simulink model "ROTATIONAL_DYNAMICS_old"  (R2024b)
settings: Solver=VariableStepAuto  StartTime=0.0  StopTime=20  RelTol=1e-3
values from neighbouring files (symbols this model uses):
  A_alt_aug = [A_alt, zeros(size(A_alt,1),1); -C_alt, 0]    [STATE_SPACE_CALCULATIONS_v2.m]
  A_altitude = [ ... (first row only)    [STATE_SPACE_CALCULATIONS.m]
  B_alt_aug = [B_alt; 0]    [STATE_SPACE_CALCULATIONS_v2.m]
  B_altitude = [ ... (first row only)    [STATE_SPACE_CALCULATIONS.m]
  C_alt_aug = [C_alt 0]    [STATE_SPACE_CALCULATIONS_v2.m]
  C_altitude = [1, 0, 0]    [STATE_SPACE_CALCULATIONS.m]
  D_alt_aug = D_alt    [STATE_SPACE_CALCULATIONS_v2.m]
  D_altitude = [0]    [STATE_SPACE_CALCULATIONS.m]
  K_alt_aug = lqr(A_alt_aug, B_alt_aug, Q_alt_aug, R_alt)    [STATE_SPACE_CALCULATIONS_v2.m]
  K_altitude = lqr(A_altitude, B_altitude, Q_altitude, R_altitude)    [STATE_SPACE_CALCULATIONS.m]
settings Model: Creator=hazza  LastModifiedBy=hazza

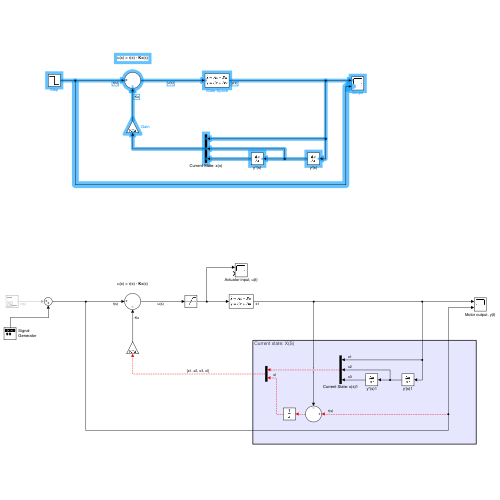
[thumbnail: Simulink's stored preview of the top-level diagram]
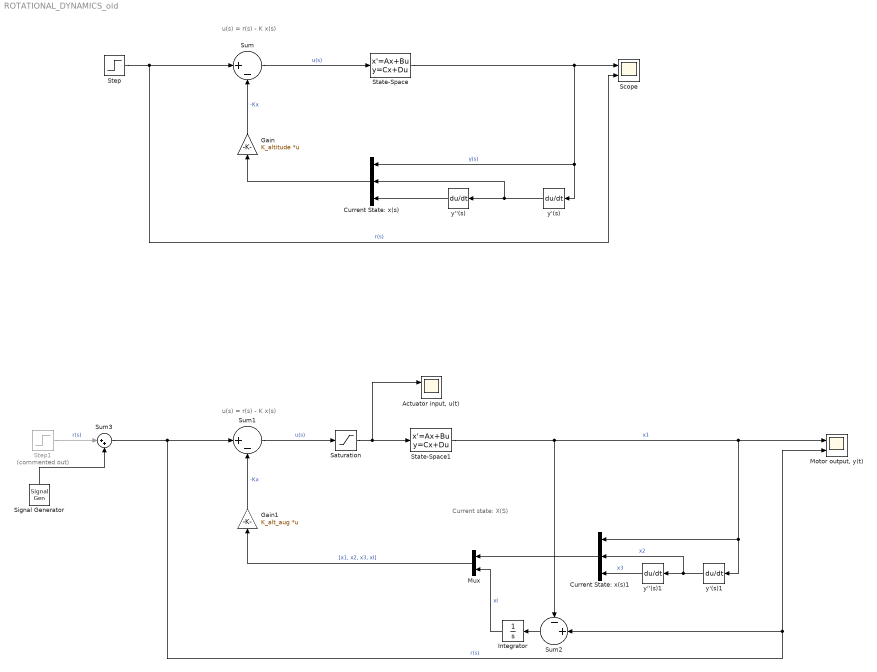
== system ROTATIONAL_DYNAMICS_old ==
  note: Current state: X(S)
  note: u(s) = r(s) - K x(s)
  note: u(s) = r(s) - K x(s)
  "Actuator input, u(t)" : Scope  NumInputPorts=2
  Current State: x(s) : Mux  Inputs=3
  Current State: x(s)1 : Mux  Inputs=3
  Gain : Gain  Gain=K_altitude  Multiplication=Matrix(K*u)
  Gain1 : Gain  Gain=K_alt_aug  Multiplication=Matrix(K*u)
  Integrator : Integrator
  "Motor output, y(t)" : Scope  NumInputPorts=2
  Mux : Mux  Inputs=2
  Saturation : Saturate  UpperLimit=95  LowerLimit=-55  ZeroCross=off
  Scope : Scope  NumInputPorts=2
  Signal Generator : SignalGenerator  Frequency=2  Units=rad/sec
  State-Space : StateSpace  A=A_altitude  B=B_altitude  C=C_altitude  D=D_altitude  InitialCondition=[0, 0, 0]
  State-Space1 : StateSpace  A=A_alt_aug  B=B_alt_aug  C=C_alt_aug  D=D_alt_aug  InitialCondition=[0, 0, 0,0]
  Step : Step  Time=10  Before=1200  After=800  SampleTime=0
  Step1 : Step  Commented=on  Time=10  Before=1200  After=800  SampleTime=0
  Sum : Sum  Inputs=|+-
  Sum1 : Sum  Inputs=|+-
  Sum2 : Sum  Inputs=-+|
  Sum3 : Sum  Inputs=|++
  y''(s) : Derivative
  y''(s)1 : Derivative
  y'(s) : Derivative
  y'(s)1 : Derivative
  wires:
  Step/1 -> Scope/2, Sum/1  "r(s)"
  Sum/1 -> State-Space/1  "u(s)"
  Gain/1 -> Sum/2  "-Kx"
  Current State: x(s)/1 -> Gain/1
  State-Space/1 -> Scope/1, y'(s)/1, Current State: x(s)/1  "y(s)"
  y'(s)/1 -> y''(s)/1, Current State: x(s)/2
  y''(s)/1 -> Current State: x(s)/3
  Gain1/1 -> Sum1/2  "-Kx"
  State-Space1/1 -> Sum2/1, "Motor output, y(t)"/1, y'(s)1/1, Current State: x(s)1/1  "x1"
  Sum3/1 -> Sum1/1, "Motor output, y(t)"/2, Sum2/2  "r(s)"
  Sum1/1 -> Saturation/1  "u(s)"
  y'(s)1/1 -> y''(s)1/1, Current State: x(s)1/2  "x2"
  Sum2/1 -> Integrator/1
  Current State: x(s)1/1 -> Mux/1
  Integrator/1 -> Mux/2  "xI"
  Mux/1 -> Gain1/1  "[x1, x2, x3, xI]"
  Saturation/1 -> "Actuator input, u(t)"/1, State-Space1/1
  Step1/1 -> Sum3/1  "r(s)"
  Signal Generator/1 -> Sum3/2
  y''(s)1/1 -> Current State: x(s)1/3  "x3"
